simulink model "Elevator_Control"  (R2020b)
settings: Solver=VariableStepAuto  StartTime=0.0  StopTime=inf  RelTol=1e-3
settings Model: EnablePacing=on  PacingRate=0.056000  Creator=vijay jagtap  LastModifiedBy=vijay jagtap

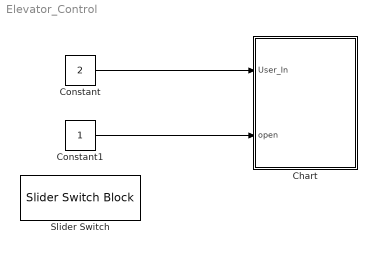
== system Elevator_Control ==
  Chart : Stateflow chart  TreatAsAtomicUnit=on
  Constant : Constant  Value=2
  Constant1 : Constant
  Slider Switch : SliderSwitchBlock
      settings: Values={{'Off', 'On'}, [0 1]}
  wires:
  Constant/1 -> Chart/1(User_In)
  Constant1/1 -> Chart/2(open)

== stateflow chart Elevator_Control/Chart ==
  state Close
  state Open
    state Ground
    state First_Floor
    state Second_Floor
    Second_Floor -> Ground [order 2] : [User_In == 0]
    (default) -> Ground
    First_Floor -> Ground [order 1] : [User_In == 0]
    Second_Floor -> First_Floor [order 1] : [User_In == 1]
    Ground -> First_Floor [order 1] : [User_In == 1]
    First_Floor -> Second_Floor [order 2] : [User_In == 2]
    Ground -> Second_Floor [order 2] : [User_In == 2]
  (default) -> Close
  Open -> Close : [open == 0]
  Close -> Open : [open == 1]
  data: User_In input; open input
